simulink model "directiondetection"  (R2020a)
settings: Solver=VariableStepAuto  StartTime=0.0  StopTime=10.0  RelTol=1e-3
libraries: simulink x1
settings Model: Creator=pc  LastModifiedBy=pc

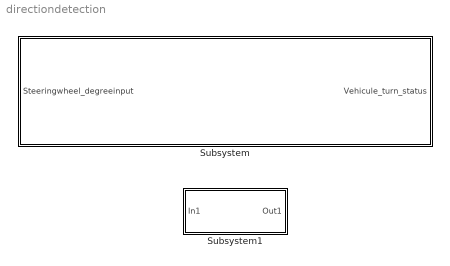
== system directiondetection ==
  Subsystem : Subsystem
  Subsystem1 : Subsystem

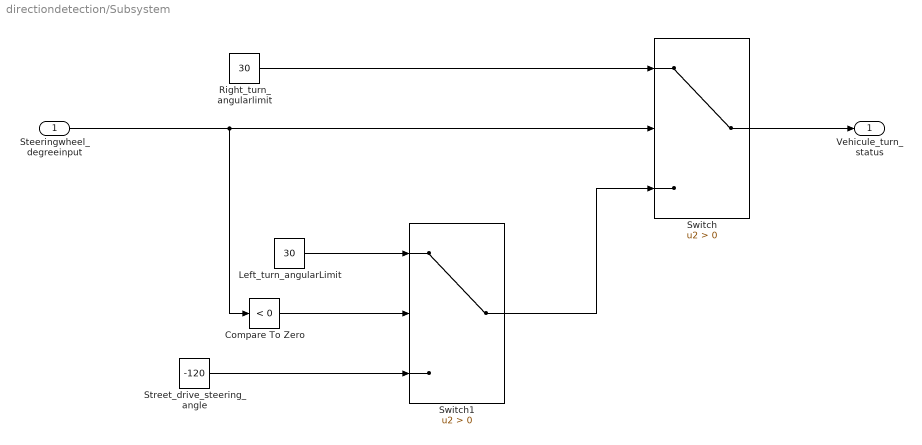
== system directiondetection/Subsystem ==
  Steeringwheel_degreeinput : Inport
  Compare To Zero : simulink/Logic and Bit Operations/Compare To Zero  relop=<  OutDataTypeStr=boolean
  Left_turn_angularLimit : Constant  Value=30
  Right_turn_angularlimit : Constant  Value=30
  Street_drive_steering_angle : Constant  Value=-120
  Switch : Switch  Criteria=u2 > Threshold
  Switch1 : Switch  Criteria=u2 > Threshold
  Vehicule_turn_status : Outport
  wires:
  Switch1/1 -> Switch/3
  Street_drive_steering_angle/1 -> Switch1/3
  Compare To Zero/1 -> Switch1/2
  Right_turn_angularlimit/1 -> Switch/1
  Left_turn_angularLimit/1 -> Switch1/1
  Switch/1 -> Vehicule_turn_status/1
  Steeringwheel_degreeinput/1 -> Compare To Zero/1, Switch/2

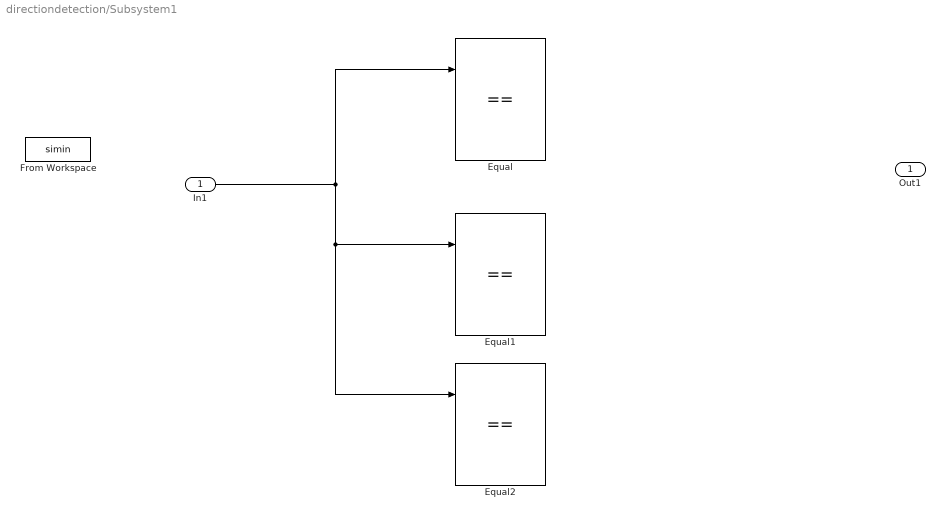
== system directiondetection/Subsystem1 ==
  In1 : Inport
  Equal : RelationalOperator  Operator===  OutDataTypeStr=boolean  RndMeth=Simplest
  Equal1 : RelationalOperator  Operator===  OutDataTypeStr=boolean  RndMeth=Simplest
  Equal2 : RelationalOperator  Operator===  OutDataTypeStr=boolean  RndMeth=Simplest
  From Workspace : FromWorkspace  VariableName=simin
  Out1 : Outport
  wires:
  In1/1 -> Equal1/1, Equal2/1, Equal/1
